simulink model "comp_curves"  (R2021b)
settings: Solver=VariableStepAuto  StartTime=0.0  StopTime=0  RelTol=1e-3
settings Model: Creator=billtubbs  LastModifiedBy=billtubbs

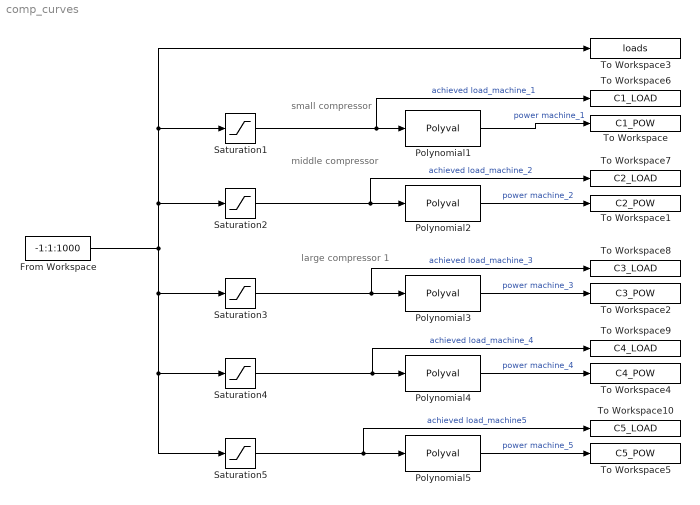
== system comp_curves ==
  note: small compressor
  note: middle compressor
  note: large compressor 1
  From Workspace : FromWorkspace  VariableName=-1:1:1000
  Polynomial1 : Polyval  Coefs=[-9e-08 4e-05 -0.0052 0.7765 15.661]
  Polynomial2 : Polyval  Coefs=[-1.42718017e-08 1.87477980e-05 -8.28649653e-03 1.88469092 -2.19952823]
  Polynomial3 : Polyval  Coefs="[-1.53490519e-09  2.28838030e-06 -9.59520873e-04 6.18821903e-01 7.51758182e+01]"
  Polynomial4 : Polyval  Coefs="[-1.53490519e-09  2.28838030e-06 -9.59520873e-04 6.18821903e-01 7.51758182e+01]"
  Polynomial5 : Polyval  Coefs="[-1.53490519e-09  2.28838030e-06 -9.59520873e-04 6.18821903e-01 7.51758182e+01]"
  Saturation1 : Saturate  UpperLimit=220  LowerLimit=56
  Saturation2 : Saturate  UpperLimit=537  LowerLimit=237
  Saturation3 : Saturate  UpperLimit=795  LowerLimit=194
  Saturation4 : Saturate  UpperLimit=795  LowerLimit=194
  Saturation5 : Saturate  UpperLimit=795  LowerLimit=194
  To Workspace : ToWorkspace  VariableName=C1_POW  SaveFormat=Timeseries  SampleTime=-1
  To Workspace1 : ToWorkspace  VariableName=C2_POW  SaveFormat=Timeseries  SampleTime=-1
  To Workspace10 : ToWorkspace  VariableName=C5_LOAD  SaveFormat=Timeseries  SampleTime=-1
  To Workspace2 : ToWorkspace  VariableName=C3_POW  SaveFormat=Timeseries  SampleTime=-1
  To Workspace3 : ToWorkspace  VariableName=loads  SaveFormat=Timeseries  SampleTime=-1
  To Workspace4 : ToWorkspace  VariableName=C4_POW  SaveFormat=Timeseries  SampleTime=-1
  To Workspace5 : ToWorkspace  VariableName=C5_POW  SaveFormat=Timeseries  SampleTime=-1
  To Workspace6 : ToWorkspace  VariableName=C1_LOAD  SaveFormat=Timeseries  SampleTime=-1
  To Workspace7 : ToWorkspace  VariableName=C2_LOAD  SaveFormat=Timeseries  SampleTime=-1
  To Workspace8 : ToWorkspace  VariableName=C3_LOAD  SaveFormat=Timeseries  SampleTime=-1
  To Workspace9 : ToWorkspace  VariableName=C4_LOAD  SaveFormat=Timeseries  SampleTime=-1
  wires:
  Saturation1/1 -> To Workspace6/1, Polynomial1/1  "achieved load_machine_1"
  From Workspace/1 -> Saturation3/1, Saturation5/1, Saturation4/1, To Workspace3/1, Saturation1/1, Saturation2/1
  Polynomial1/1 -> To Workspace/1  "power machine_1"
  Saturation2/1 -> To Workspace7/1, Polynomial2/1  "achieved load_machine_2"
  Polynomial2/1 -> To Workspace1/1  "power machine_2"
  Saturation3/1 -> To Workspace8/1, Polynomial3/1  "achieved load_machine_3"
  Polynomial3/1 -> To Workspace2/1  "power machine_3"
  Saturation4/1 -> To Workspace9/1, Polynomial4/1  "achieved load_machine_4"
  Polynomial4/1 -> To Workspace4/1  "power machine_4"
  Saturation5/1 -> To Workspace10/1, Polynomial5/1  "achieved load_machine5"
  Polynomial5/1 -> To Workspace5/1  "power machine_5"
